simulink model "PHRI_MODEL_PROJECT"  (R2020b)
settings: Solver=VariableStepAuto  StartTime=0.0  StopTime=20  RelTol=1e-3
values from neighbouring files (symbols this model uses):
  A = [1 Ts;0 1]    [parameters.m]
  Be = 1    [parameters.m]
  beta = 2*pi*Fc*Ts / (1+2*pi*Fc*Ts)    (= 0.111635211705)    [parameters.m]
  Bh = 0.02    [parameters.m]
  Bh_hat = 0.05    [parameters.m]
  C = [1 0]    [parameters.m]
  delayCommM2S = 400    [parameters.m]
  delayCommS2M = 400    [parameters.m]
  Fc = 20    [parameters.m]
  Fc_h = 1    [parameters.m]
  Jh = 0.00002    (= 2e-05)    [parameters.m]
  k_m = 19.34    [parameters.m]
  k_s = 19.34    [parameters.m]
  Kc2v_m = 2    [parameters.m]
  Kc2v_s = 2    [parameters.m]
  Kd_h = 1.125    [parameters.m]
  Kd_m = 1.5    [parameters.m]
  Kd_s = 1.5    [parameters.m]
  Ke = 10    [parameters.m]
  Kh_hat = 1    [parameters.m]
  Kh_max = 50    [parameters.m]
  Kp_h = 1    [parameters.m]
  Kp_m = 1    [parameters.m]
  Kp_s = 1    [parameters.m]
  Kt2c_m = 1.182    [parameters.m]
  Kt2c_s = 1.182    [parameters.m]
  lArm_m = 0.1    [parameters.m]
  lArm_s = 0.1    [parameters.m]
  maxCurrent_m = 4.5    [parameters.m]
  maxCurrent_s = 4.5    [parameters.m]
  PosRef = 1    [parameters.m]
  qe = 2    [parameters.m]
  stopTime = str2double(stopTime)    [parameters.m]
  tau_m = 1.217    [parameters.m]
  tau_s = 1.217    [parameters.m]
  Ts = 0.001    [parameters.m]
  Variance = 0.0000001    (= 1e-07)    [parameters.m]
undefined symbols (not defined in the file or in its folder): DiscIntNeverNeededParam, Discrete, Time
libraries: simulink_extras x37, dspsigops x37, ctrlSharedLib x16, cstblocks x1
(part 2 of 3)

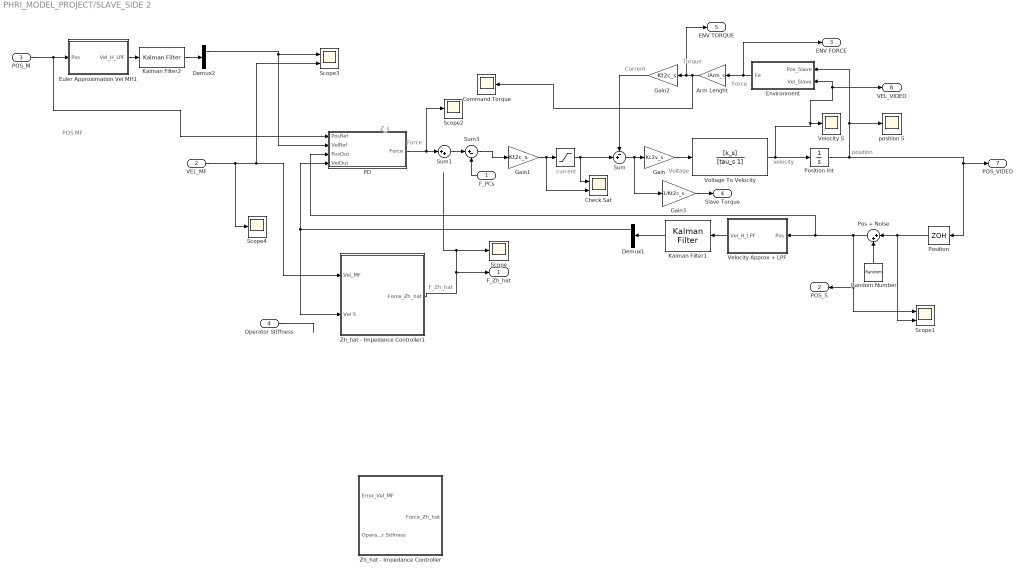
== system PHRI_MODEL_PROJECT/SLAVE_SIDE 2 ==
  note: POS MF
  note: current
  note: Force
  note: velocity
  note: position
  note: Current
  note: Voltage
  note: Torque
  note: Z_s
  note: Force
  note: F_Zh_hat
  F_PCs : Inport
  VEL_MF : Inport  Port=2
  POS_M : Inport  Port=3
  Operator Stiffness : Inport  Port=4
  " " : Saturate  UpperLimit=maxCurrent_s  LowerLimit=-maxCurrent_s
  Arm Lenght : Gain  Gain=lArm_s
  Check Sat : Scope  NumInputPorts=2
  Command Torque : Scope
  Demux1 : Demux  Outputs=2
  Demux2 : Demux  Outputs=2
  "Environment " : Subsystem
  Euler Approximation Vel MH1 : Subsystem
  Gain : Gain  Gain=Kc2v_s
  Gain1 : Gain  Gain=Kt2c_s
  Gain2 : Gain  Gain=Kt2c_s
  Gain3 : Gain  Gain=1/Kt2c_s
  Kalman Filter1 : ctrlSharedLib/Kalman Filter  TimeDomain=Discrete-Time  UseCurrentEstimator=off  ModelSource=Individual A, B, C, D matrices  ModelSourceVariable=ss(A,0,C,0)  A=A  B=1  C=C  D=0  NumberOfStates=2  NumberOfInputs=1  NumberOfOutputs=1  InitialEstimateSource=Dialog  X0=0  P0=10  UseK=off  UseGH=off  NumberOfProcessNoiseInputs=1  G=1  TimeInvariantG=on  H=0  TimeInvariantH=on  Q=0.05  TimeInvariantQ=on  R=1  TimeInvariantR=on  N=0  TimeInvariantN=on  AddInputPort=off  AddEnablePort=off  OutputEstimatedY=off  OutputP=off  Ts=Ts
  Kalman Filter2 : ctrlSharedLib/Kalman Filter  TimeDomain=Discrete-Time  UseCurrentEstimator=off  ModelSource=Individual A, B, C, D matrices  ModelSourceVariable=ss(A,0,C,0)  A=A  B=1  C=C  D=0  NumberOfStates=2  NumberOfInputs=1  NumberOfOutputs=1  InitialEstimateSource=Dialog  X0=0  P0=10  UseK=off  UseGH=off  NumberOfProcessNoiseInputs=1  G=1  TimeInvariantG=on  H=0  TimeInvariantH=on  Q=0.05  TimeInvariantQ=on  R=1  TimeInvariantR=on  N=0  TimeInvariantN=on  AddInputPort=off  AddEnablePort=off  OutputEstimatedY=off  OutputP=off  Ts=Ts
  PD : Subsystem
  Pos + Noise : Sum  Inputs=|++
  Position : ZeroOrderHold  SampleTime=Ts
  "Position Int " : Integrator
  Random Number : RandomNumber  Variance=Variance  SampleTime=Ts
  Scope : Scope
  Scope1 : Scope  NumInputPorts=2
  Scope2 : Scope
  Scope3 : Scope  NumInputPorts=2
  Scope4 : Scope
  Sum : Sum  Inputs=-+|
  Sum1 : Sum  Inputs=|++
  Sum3 : Sum  Inputs=|+-
  "Velocity Approx + LPF " : Subsystem
  Velocity S : Scope
  "Voltage To Velocity " : TransferFcn  Numerator=[k_s]  Denominator=[tau_s 1]
  Zh_hat - Impedance Controller : Subsystem
  Zh_hat - Impedance Controller1 : Subsystem
  "position S " : Scope
  F_Zh_hat : Outport
  POS_S : Outport  Port=2
  ENV FORCE : Outport  Port=3
  Slave Torque : Outport  Port=4
  ENV TORQUE : Outport  Port=5
  VEL_VIDEO : Outport  Port=6
  POS_VIDEO : Outport  Port=7
  wires:
  PD/1(Force) -> Scope2/1, Sum1/1
  "Position Int "/1 -> Position/1, POS_VIDEO/1, "position S "/1, "Environment "/1(Pos_Slave)
  Gain1/1 -> Check Sat/2, " "/1
  Gain2/1 -> Sum/1
  "Environment "/1(Fe) -> ENV FORCE/1, Arm Lenght/1
  "Voltage To Velocity "/1 -> "Position Int "/1, Velocity S/1, "Environment "/2("Vel_Slave "), VEL_VIDEO/1
  Sum/1 -> Gain3/1, Gain/1
  Gain/1 -> "Voltage To Velocity "/1
  Sum1/1 -> Sum3/1
  " "/1 -> Check Sat/1, Sum/2
  Arm Lenght/1 -> Command Torque/1, ENV TORQUE/1, Gain2/1
  Zh_hat - Impedance Controller1/1("Force_Zh_hat ") -> Scope/1, F_Zh_hat/1
  F_PCs/1 -> Sum3/2
  Operator Stiffness/1 -> ?
  VEL_MF/1 -> Scope4/1, Scope3/2, Zh_hat - Impedance Controller1/1(Vel_MF)
  Pos + Noise/1 -> PD/3(PosOut), "Velocity Approx + LPF "/1(Pos), POS_S/1, Scope1/1
  Random Number/1 -> Pos + Noise/2
  Demux1/1 -> PD/4(VelOut), Zh_hat - Impedance Controller1/2(Vel S)
  Position/1 -> Scope1/2, Pos + Noise/1
  "Velocity Approx + LPF "/1("Vel_H_LPF ") -> Kalman Filter1/1
  Kalman Filter1/1 -> Demux1/1
  Gain3/1 -> Slave Torque/1
  POS_M/1 -> PD/1(PosRef), Euler Approximation Vel MH1/1(Pos)
  Euler Approximation Vel MH1/1("Vel_H_LPF ") -> Kalman Filter2/1
  Kalman Filter2/1 -> Demux2/1
  Demux2/1 -> PD/2(VelRef), Scope3/1
  Sum3/1 -> Gain1/1

== system PHRI_MODEL_PROJECT/Velocity Approx + LPF 3 ==
  Pos : Inport
  Constant : Constant  Value=Ts  SampleTime=Ts
  Constant1 : Constant  Value=beta
  "Euler Approximation " : MATLAB Function  TreatAsAtomicUnit=on
  Unit Delay : UnitDelay  SampleTime=Ts  HasFrameUpgradeWarning=on
  Unit Delay1 : UnitDelay  SampleTime=Ts  HasFrameUpgradeWarning=on
  "Vel_H_LPF " : Outport
  wires:
  Pos/1 -> Unit Delay/1, "Euler Approximation "/3(pos)
  Constant/1 -> "Euler Approximation "/2(Ts)
  Unit Delay/1 -> "Euler Approximation "/4(posPrev)
  Unit Delay1/1 -> "Euler Approximation "/5(filteredPrev)
  "Euler Approximation "/1(filtered) -> Unit Delay1/1, "Vel_H_LPF "/1
  Constant1/1 -> "Euler Approximation "/1(beta)

== system PHRI_MODEL_PROJECT/MASTER SIDE/Intentional operator force ==
  Pos Ref : Inport
  Vel Ref : Inport  Port=2
  Pos Slave : Inport  Port=3
  Vel Slave : Inport  Port=4
  Gain : Gain  Gain=Kp_h
  Gain1 : Gain  Gain=Kd_h
  Sum : Sum
  Sum1 : Sum  Inputs=+-
  Sum2 : Sum  Inputs=+-
  "Fh_star " : Outport
  wires:
  Sum/1 -> "Fh_star "/1
  Pos Ref/1 -> Sum1/1
  Pos Slave/1 -> Sum1/2
  Vel Ref/1 -> Sum2/1
  Vel Slave/1 -> Sum2/2
  Sum1/1 -> Gain/1
  Sum2/1 -> Gain1/1
  Gain1/1 -> Sum/2
  Gain/1 -> Sum/1

== system PHRI_MODEL_PROJECT/MASTER SIDE/Operator - Dynamic model ==
  "Velocity master " : Inport
  Derivative : Derivative  CoefficientInTFapproximation=0.01
  Friction : Gain  Gain=Bh
  Inertia : Gain  Gain=Jh
  Integrator : Integrator
  "Stiffness " : Gain  Gain=Kh_hat
  Sum : Sum  Inputs=+++
  Force : Outport
  wires:
  "Velocity master "/1 -> Friction/1, Integrator/1, Derivative/1
  Derivative/1 -> Inertia/1
  Inertia/1 -> Sum/2
  Friction/1 -> Sum/1
  Sum/1 -> Force/1
  Integrator/1 -> "Stiffness "/1
  "Stiffness "/1 -> ?

== system PHRI_MODEL_PROJECT/MASTER SIDE/Velocity Approx + LPF 3 ==
  Pos : Inport
  Constant : Constant  Value=Ts  SampleTime=Ts
  Constant1 : Constant  Value=beta
  "Euler Approximation " : MATLAB Function  TreatAsAtomicUnit=on
  Unit Delay : UnitDelay  SampleTime=Ts  HasFrameUpgradeWarning=on
  Unit Delay1 : UnitDelay  SampleTime=Ts  HasFrameUpgradeWarning=on
  "Vel_H_LPF " : Outport
  wires:
  Pos/1 -> Unit Delay/1, "Euler Approximation "/3(pos)
  Constant/1 -> "Euler Approximation "/2(Ts)
  Unit Delay/1 -> "Euler Approximation "/4(posPrev)
  Unit Delay1/1 -> "Euler Approximation "/5(filteredPrev)
  "Euler Approximation "/1(filtered) -> Unit Delay1/1, "Vel_H_LPF "/1
  Constant1/1 -> "Euler Approximation "/1(beta)

== system PHRI_MODEL_PROJECT/MASTER SIDE1/Euler Approximation Vel MH2 ==
  Pos : Inport
  Clock : simulink_extras/Flip Flops/Clock  period=Ts*2
  Clock1 : simulink_extras/Flip Flops/Clock  period=Ts*2
  Constant : Constant  Value=Ts
  Constant1 : Constant  Value=beta
  "Euler Approximation " : MATLAB Function  TreatAsAtomicUnit=on
  Sample and Hold : dspsigops/Sample and Hold  trig=Rising edge  initCond=0  latchinput=on
  Sample and Hold1 : dspsigops/Sample and Hold  trig=Rising edge  initCond=0  latchinput=on
  "Vel_H_LPF " : Outport
  wires:
  Pos/1 -> Sample and Hold/1, "Euler Approximation "/3(pos)
  Constant/1 -> "Euler Approximation "/2(Ts)
  Sample and Hold/1 -> "Euler Approximation "/4(posPrev)
  Clock/1 -> Sample and Hold/Trigger
  Sample and Hold1/1 -> "Euler Approximation "/5(filteredPrev)
  "Euler Approximation "/1(filtered) -> "Vel_H_LPF "/1, Sample and Hold1/1
  Clock1/1 -> Sample and Hold1/Trigger
  Constant1/1 -> "Euler Approximation "/1(beta)

== system PHRI_MODEL_PROJECT/MASTER SIDE1/Intentional operator force ==
  Pos Ref : Inport
  Vel Ref : Inport  Port=2
  Pos Slave : Inport  Port=3
  Vel Slave : Inport  Port=4
  Gain : Gain  Gain=Kp_h
  Gain1 : Gain  Gain=Kd_h
  Sum : Sum
  Sum1 : Sum  Inputs=+-
  Sum2 : Sum  Inputs=+-
  "Fh_star " : Outport
  wires:
  Sum/1 -> "Fh_star "/1
  Pos Ref/1 -> Sum1/1
  Pos Slave/1 -> Sum1/2
  Vel Ref/1 -> Sum2/1
  Vel Slave/1 -> Sum2/2
  Sum1/1 -> Gain/1
  Sum2/1 -> Gain1/1
  Gain1/1 -> Sum/2
  Gain/1 -> Sum/1

== system PHRI_MODEL_PROJECT/MASTER SIDE1/Subsystem ==
  "Velocità " : Inport
  Derivative : Derivative  CoefficientInTFapproximation=0.01
  Friction : Gain  Gain=Bh
  Inertia : Gain  Gain=Jh
  Integrator : Integrator
  "Stiffness " : Gain  Gain=Kh_hat
  Sum : Sum  Inputs=+++
  Force : Outport
  wires:
  "Velocità "/1 -> Friction/1, Integrator/1, Derivative/1
  Derivative/1 -> Inertia/1
  Inertia/1 -> Sum/2
  Friction/1 -> Sum/1
  Sum/1 -> Force/1
  Integrator/1 -> "Stiffness "/1
  "Stiffness "/1 -> ?

== system PHRI_MODEL_PROJECT/MASTER SIDE1/Velocity Approx + LPF  ==
  Pos : Inport
  Clock : simulink_extras/Flip Flops/Clock  period=Ts*2
  Clock1 : simulink_extras/Flip Flops/Clock  period=Ts*2
  Constant : Constant  Value=Ts
  Constant1 : Constant  Value=beta
  "Euler Approximation " : MATLAB Function  TreatAsAtomicUnit=on
  Sample and Hold : dspsigops/Sample and Hold  trig=Rising edge  initCond=0  latchinput=on
  Sample and Hold1 : dspsigops/Sample and Hold  trig=Rising edge  initCond=0  latchinput=on
  "Vel_H_LPF " : Outport
  wires:
  Pos/1 -> Sample and Hold/1, "Euler Approximation "/3(pos)
  Constant/1 -> "Euler Approximation "/2(Ts)
  Sample and Hold/1 -> "Euler Approximation "/4(posPrev)
  Clock/1 -> Sample and Hold/Trigger
  Sample and Hold1/1 -> "Euler Approximation "/5(filteredPrev)
  "Euler Approximation "/1(filtered) -> "Vel_H_LPF "/1, Sample and Hold1/1
  Clock1/1 -> Sample and Hold1/Trigger
  Constant1/1 -> "Euler Approximation "/1(beta)

== system PHRI_MODEL_PROJECT/MASTER SIDE1/Virtual Coupling ==
  Pos Master : Inport
  Vel Master : Inport  Port=2
  Pos Slave : Inport  Port=3
  Vel Slave : Inport  Port=4
  Gain : Gain  Gain=Kp_m
  Gain1 : Gain  Gain=Kd_m
  Sum : Sum
  Sum1 : Sum  Inputs=-+
  Sum2 : Sum  Inputs=-+
  "F Env Virt " : Outport
  wires:
  Gain/1 -> Sum/1
  Gain1/1 -> Sum/2
  Sum2/1 -> Gain1/1
  Sum1/1 -> Gain/1
  Vel Slave/1 -> Sum2/2
  Vel Master/1 -> Sum2/1
  Pos Slave/1 -> Sum1/2
  Pos Master/1 -> Sum1/1
  Sum/1 -> "F Env Virt "/1

== system PHRI_MODEL_PROJECT/MASTER SIDE2/Intentional operator force ==
  Pos Ref : Inport
  Vel Ref : Inport  Port=2
  Pos Slave : Inport  Port=3
  Vel Slave : Inport  Port=4
  Gain : Gain  Gain=Kp_h
  Gain1 : Gain  Gain=Kd_h
  Sum : Sum
  Sum1 : Sum  Inputs=+-
  Sum2 : Sum  Inputs=+-
  "Fh_star " : Outport
  wires:
  Sum/1 -> "Fh_star "/1
  Pos Ref/1 -> Sum1/1
  Pos Slave/1 -> Sum1/2
  Vel Ref/1 -> Sum2/1
  Vel Slave/1 -> Sum2/2
  Sum1/1 -> Gain/1
  Sum2/1 -> Gain1/1
  Gain1/1 -> Sum/2
  Gain/1 -> Sum/1

== system PHRI_MODEL_PROJECT/MASTER SIDE2/Subsystem ==
  "Velocità " : Inport
  Derivative : Derivative  CoefficientInTFapproximation=0.01
  Friction : Gain  Gain=Bh
  Inertia : Gain  Gain=Jh
  Integrator : Integrator
  "Stiffness " : Gain  Gain=Kh_hat
  Sum : Sum  Inputs=+++
  Force : Outport
  wires:
  "Velocità "/1 -> Friction/1, Integrator/1, Derivative/1
  Derivative/1 -> Inertia/1
  Inertia/1 -> Sum/2
  Friction/1 -> Sum/1
  Sum/1 -> Force/1
  Integrator/1 -> "Stiffness "/1
  "Stiffness "/1 -> ?

== system PHRI_MODEL_PROJECT/MASTER SIDE2/Velocity Approx + LPF  ==
  Pos : Inport
  Clock : simulink_extras/Flip Flops/Clock  period=Ts*2
  Clock1 : simulink_extras/Flip Flops/Clock  period=Ts*2
  Constant : Constant  Value=Ts
  Constant1 : Constant  Value=beta
  "Euler Approximation " : MATLAB Function  TreatAsAtomicUnit=on
  Sample and Hold : dspsigops/Sample and Hold  trig=Rising edge  initCond=0  latchinput=on
  Sample and Hold1 : dspsigops/Sample and Hold  trig=Rising edge  initCond=0  latchinput=on
  "Vel_H_LPF " : Outport
  wires:
  Pos/1 -> Sample and Hold/1, "Euler Approximation "/3(pos)
  Constant/1 -> "Euler Approximation "/2(Ts)
  Sample and Hold/1 -> "Euler Approximation "/4(posPrev)
  Clock/1 -> Sample and Hold/Trigger
  Sample and Hold1/1 -> "Euler Approximation "/5(filteredPrev)
  "Euler Approximation "/1(filtered) -> "Vel_H_LPF "/1, Sample and Hold1/1
  Clock1/1 -> Sample and Hold1/Trigger
  Constant1/1 -> "Euler Approximation "/1(beta)

== system PHRI_MODEL_PROJECT/MASTER SIDE2/Velocity Approx + LPF 1 ==
  Pos : Inport
  Clock : simulink_extras/Flip Flops/Clock  period=Ts*2
  Clock1 : simulink_extras/Flip Flops/Clock  period=Ts*2
  Constant : Constant  Value=Ts
  Constant1 : Constant  Value=beta
  "Euler Approximation " : MATLAB Function  TreatAsAtomicUnit=on
  Sample and Hold : dspsigops/Sample and Hold  trig=Rising edge  initCond=0  latchinput=on
  Sample and Hold1 : dspsigops/Sample and Hold  trig=Rising edge  initCond=0  latchinput=on
  "Vel_H_LPF " : Outport
  wires:
  Pos/1 -> Sample and Hold/1, "Euler Approximation "/3(pos)
  Constant/1 -> "Euler Approximation "/2(Ts)
  Sample and Hold/1 -> "Euler Approximation "/4(posPrev)
  Clock/1 -> Sample and Hold/Trigger
  Sample and Hold1/1 -> "Euler Approximation "/5(filteredPrev)
  "Euler Approximation "/1(filtered) -> "Vel_H_LPF "/1, Sample and Hold1/1
  Clock1/1 -> Sample and Hold1/Trigger
  Constant1/1 -> "Euler Approximation "/1(beta)

== system PHRI_MODEL_PROJECT/MASTER SIDE2/Velocity Approx + LPF 2 ==
  Pos : Inport
  Clock : simulink_extras/Flip Flops/Clock  period=Ts*2
  Clock1 : simulink_extras/Flip Flops/Clock  period=Ts*2
  Constant : Constant  Value=Ts
  Constant1 : Constant  Value=beta
  "Euler Approximation " : MATLAB Function  TreatAsAtomicUnit=on
  Sample and Hold : dspsigops/Sample and Hold  trig=Rising edge  initCond=0  latchinput=on
  Sample and Hold1 : dspsigops/Sample and Hold  trig=Rising edge  initCond=0  latchinput=on
  "Vel_H_LPF " : Outport
  wires:
  Pos/1 -> Sample and Hold/1, "Euler Approximation "/3(pos)
  Constant/1 -> "Euler Approximation "/2(Ts)
  Sample and Hold/1 -> "Euler Approximation "/4(posPrev)
  Clock/1 -> Sample and Hold/Trigger
  Sample and Hold1/1 -> "Euler Approximation "/5(filteredPrev)
  "Euler Approximation "/1(filtered) -> "Vel_H_LPF "/1, Sample and Hold1/1
  Clock1/1 -> Sample and Hold1/Trigger
  Constant1/1 -> "Euler Approximation "/1(beta)

== system PHRI_MODEL_PROJECT/MASTER SIDE2/Velocity Approx + LPF 3 ==
  Pos : Inport
  Clock : simulink_extras/Flip Flops/Clock  period=Ts*2
  Clock1 : simulink_extras/Flip Flops/Clock  period=Ts*2
  Constant : Constant  Value=Ts
  Constant1 : Constant  Value=beta
  "Euler Approximation " : MATLAB Function  TreatAsAtomicUnit=on
  Sample and Hold : dspsigops/Sample and Hold  trig=Rising edge  initCond=0  latchinput=on
  Sample and Hold1 : dspsigops/Sample and Hold  trig=Rising edge  initCond=0  latchinput=on
  "Vel_H_LPF " : Outport
  wires:
  Pos/1 -> Sample and Hold/1, "Euler Approximation "/3(pos)
  Constant/1 -> "Euler Approximation "/2(Ts)
  Sample and Hold/1 -> "Euler Approximation "/4(posPrev)
  Clock/1 -> Sample and Hold/Trigger
  Sample and Hold1/1 -> "Euler Approximation "/5(filteredPrev)
  "Euler Approximation "/1(filtered) -> "Vel_H_LPF "/1, Sample and Hold1/1
  Clock1/1 -> Sample and Hold1/Trigger
  Constant1/1 -> "Euler Approximation "/1(beta)

== system PHRI_MODEL_PROJECT/POPC - Master Side/PC - Master side ==
  E_PO - Master : Inport
  "Velocity Master " : Inport  Port=2
  E_POm : Scope
  E_POm1 : Scope
  PASSIVE CONTROLLER PCm : MATLAB Function  TreatAsAtomicUnit=on
  Unit Delay : UnitDelay  SampleTime=Ts  HasFrameUpgradeWarning=on
  dt : Constant  Value=Ts
  ALPHA : Outport
  Energy PCm : Outport  Port=2
  wires:
  Unit Delay/1 -> Energy PCm/1, PASSIVE CONTROLLER PCm/4(E_PCm_prev)
  dt/1 -> PASSIVE CONTROLLER PCm/2(Ts)
  E_PO - Master/1 -> E_POm/1, PASSIVE CONTROLLER PCm/1(E_POm)
  PASSIVE CONTROLLER PCm/1(E_PCm) -> Unit Delay/1
  PASSIVE CONTROLLER PCm/2(alpha_m) -> E_POm1/1, ALPHA/1
  "Velocity Master "/1 -> PASSIVE CONTROLLER PCm/3(v_m)

== system PHRI_MODEL_PROJECT/POPC - Master Side/PO Input - Slave to Master (Cause) ==
  Force_Env : Inport
  Velocity Master Delayed : Inport  Port=2
  E_Rin : Scope
  PASSIVE OBSERVER S2M E Right INPUT : Subsystem
  Input Energy : Outport
  wires:
  PASSIVE OBSERVER S2M E Right INPUT/1(E-Rin) -> Input Energy/1, E_Rin/1
  Velocity Master Delayed/1 -> PASSIVE OBSERVER S2M E Right INPUT/2("Vel_M ")
  Force_Env/1 -> PASSIVE OBSERVER S2M E Right INPUT/1(Env_Force)

== system PHRI_MODEL_PROJECT/POPC - Master Side/PO Output - Master to Slave (Effect) ==
  note: E Left Out
  Velocity Master : Inport
  Force Env Delayed : Inport  Port=2
  E_Lout : Scope
  PASSIVE OBSERVER M2S E Left OUTPUT : Subsystem
  Output energy : Outport
  wires:
  Velocity Master/1 -> PASSIVE OBSERVER M2S E Left OUTPUT/1(Velocity Master)
  PASSIVE OBSERVER M2S E Left OUTPUT/1(E-Lout) -> Output energy/1, E_Lout/1
  Force Env Delayed/1 -> PASSIVE OBSERVER M2S E Left OUTPUT/2(Force Env Delayed)

== system PHRI_MODEL_PROJECT/POPC - Master Side1/PC - Master side ==
  E_PO - Master : Inport
  "Velocity Master " : Inport  Port=2
  Clock : simulink_extras/Flip Flops/Clock  period=Ts*2
  E_POm : Scope
  PASSIVE CONTROLLER PCm : MATLAB Function  TreatAsAtomicUnit=on
  Sample and Hold : dspsigops/Sample and Hold  trig=Rising edge  initCond=0  latchinput=on
  dt : Constant  Value=Ts
  ALPHA : Outport
  Energy PCm : Outport  Port=2
  wires:
  Sample and Hold/1 -> PASSIVE CONTROLLER PCm/4(E_PCm_prev)
  dt/1 -> PASSIVE CONTROLLER PCm/2(dt)
  E_PO - Master/1 -> E_POm/1, PASSIVE CONTROLLER PCm/1(E_POm)
  Clock/1 -> Sample and Hold/Trigger
  PASSIVE CONTROLLER PCm/1(E_PCm) -> Sample and Hold/1, Energy PCm/1
  PASSIVE CONTROLLER PCm/2(alpha_m) -> ALPHA/1
  "Velocity Master "/1 -> PASSIVE CONTROLLER PCm/3(v_m)

== system PHRI_MODEL_PROJECT/POPC - Master Side1/PO Input - Slave to Master (Cause) ==
  Force_Env : Inport
  Velocity Master Delayed : Inport  Port=2
  E_Rin : Scope
  PASSIVE OBSERVER S2M E Right INPUT : Subsystem
  Input Energy : Outport
  wires:
  PASSIVE OBSERVER S2M E Right INPUT/1(E-Rin) -> Input Energy/1, E_Rin/1
  Velocity Master Delayed/1 -> PASSIVE OBSERVER S2M E Right INPUT/2("Vel_M ")
  Force_Env/1 -> PASSIVE OBSERVER S2M E Right INPUT/1(Env_Force)

== system PHRI_MODEL_PROJECT/POPC - Master Side1/PO Output - Master to Slave (Effect) ==
  note: E Left Out
  Velocity Master : Inport
  Force Env Delayed : Inport  Port=2
  E_Lout : Scope
  PASSIVE OBSERVER M2S E Left OUTPUT : Subsystem
  Output energy : Outport
  wires:
  Velocity Master/1 -> PASSIVE OBSERVER M2S E Left OUTPUT/1(Velocity Master)
  PASSIVE OBSERVER M2S E Left OUTPUT/1(E-Lout) -> Output energy/1, E_Lout/1
  Force Env Delayed/1 -> PASSIVE OBSERVER M2S E Left OUTPUT/2(Force Env Delayed)

== system PHRI_MODEL_PROJECT/POPC - Master Side2/PC - Master side ==
  E_PO - Master : Inport
  "Velocity Master " : Inport  Port=2
  Clock : simulink_extras/Flip Flops/Clock  period=Ts*2
  E_POm : Scope
  PASSIVE CONTROLLER PCm : MATLAB Function  TreatAsAtomicUnit=on
  Sample and Hold : dspsigops/Sample and Hold  trig=Rising edge  initCond=0  latchinput=on
  dt : Constant  Value=Ts
  ALPHA : Outport
  Energy PCm : Outport  Port=2
  wires:
  Sample and Hold/1 -> PASSIVE CONTROLLER PCm/4(E_PCm_prev)
  dt/1 -> PASSIVE CONTROLLER PCm/2(dt)
  E_PO - Master/1 -> E_POm/1, PASSIVE CONTROLLER PCm/1(E_POm)
  Clock/1 -> Sample and Hold/Trigger
  PASSIVE CONTROLLER PCm/1(E_PCm) -> Sample and Hold/1, Energy PCm/1
  PASSIVE CONTROLLER PCm/2(alpha_m) -> ALPHA/1
  "Velocity Master "/1 -> PASSIVE CONTROLLER PCm/3(v_m)

== system PHRI_MODEL_PROJECT/POPC - Master Side2/PO Input - Slave to Master (Cause) ==
  Force_Env : Inport
  Velocity Master Delayed : Inport  Port=2
  E_Rin : Scope
  PASSIVE OBSERVER S2M E Right INPUT : Subsystem
  Input Energy : Outport
  wires:
  PASSIVE OBSERVER S2M E Right INPUT/1(E-Rin) -> Input Energy/1, E_Rin/1
  Velocity Master Delayed/1 -> PASSIVE OBSERVER S2M E Right INPUT/2("Vel_M ")
  Force_Env/1 -> PASSIVE OBSERVER S2M E Right INPUT/1(Env_Force)

== system PHRI_MODEL_PROJECT/POPC - Master Side2/PO Output - Master to Slave (Effect) ==
  note: E Left Out
  Velocity Master : Inport
  Force Env Delayed : Inport  Port=2
  E_Lout : Scope
  PASSIVE OBSERVER M2S E Left OUTPUT : Subsystem
  Output energy : Outport
  wires:
  Velocity Master/1 -> PASSIVE OBSERVER M2S E Left OUTPUT/1(Velocity Master)
  PASSIVE OBSERVER M2S E Left OUTPUT/1(E-Lout) -> Output energy/1, E_Lout/1
  Force Env Delayed/1 -> PASSIVE OBSERVER M2S E Left OUTPUT/2(Force Env Delayed)

== system PHRI_MODEL_PROJECT/POPC - Slave Side/PASSIVE OBSERVER Left Input ==
  Force Env Delayed : Inport
  Velocity Master : Inport  Port=2
  Add : Sum
  Product : Product
  Unit Delay : UnitDelay  SampleTime=Ts  HasFrameUpgradeWarning=on
  E-Lin : Outport
  wires:
  Velocity Master/1 -> Product/1
  Force Env Delayed/1 -> Product/2
  Product/1 -> Add/2
  Unit Delay/1 -> Add/1
  Add/1 -> Unit Delay/1, E-Lin/1

== system PHRI_MODEL_PROJECT/POPC - Slave Side/PASSIVE OBSERVER Right Output ==
  Force Env : Inport
  Velocity Master delayed : Inport  Port=2
  Add : Sum
  Product : Product
  Unit Delay : UnitDelay  SampleTime=Ts  HasFrameUpgradeWarning=on
  E-Rout : Outport
  wires:
  Velocity Master delayed/1 -> Product/1
  Force Env/1 -> Product/2
  Product/1 -> Add/2
  Unit Delay/1 -> Add/1
  Add/1 -> Unit Delay/1, E-Rout/1

== system PHRI_MODEL_PROJECT/POPC - Slave Side/PC Slave ==
  Energy POs : Inport
  Velocity Slave : Inport  Port=2
  Clock1 : simulink_extras/Flip Flops/Clock  period=Ts
  PASSIVE CONTROLLER PCs : MATLAB Function  TreatAsAtomicUnit=on
  Sample and Hold1 : dspsigops/Sample and Hold  trig=Rising edge  initCond=0  latchinput=on
  Scope : Scope
  Scope1 : Scope  NumInputPorts=3
  Unit Delay : UnitDelay  SampleTime=Ts  HasFrameUpgradeWarning=on
  dt1 : Constant  Value=Ts
  Energy PC : Outport
  ALPHA : Outport  Port=2
  wires:
  PASSIVE CONTROLLER PCs/1(E_PCs) -> Unit Delay/1, Scope1/3
  dt1/1 -> PASSIVE CONTROLLER PCs/3(Ts)
  PASSIVE CONTROLLER PCs/2(alpha_s) -> ALPHA/1
  Energy POs/1 -> Scope1/1, Scope/1, PASSIVE CONTROLLER PCs/2(E_POs)
  Unit Delay/1 -> Scope1/2, Energy PC/1, PASSIVE CONTROLLER PCs/1(E_PCs_prev)
  Velocity Slave/1 -> PASSIVE CONTROLLER PCs/4(v_s)
  Clock1/1 -> Sample and Hold1/Trigger

== system PHRI_MODEL_PROJECT/POPC - Slave Side1/PASSIVE OBSERVER Left Input ==
  Force Impedance Delayed : Inport
  Velocity MF : Inport  Port=2
  Add : Sum
  Clock : simulink_extras/Flip Flops/Clock  period=Ts*2
  Product : Product
  Sample and Hold : dspsigops/Sample and Hold  trig=Rising edge  initCond=0  latchinput=on
  E-Lin : Outport
  wires:
  Velocity MF/1 -> Product/1
  Force Impedance Delayed/1 -> Product/2
  Product/1 -> Add/2
  Sample and Hold/1 -> Add/1
  Add/1 -> Sample and Hold/1, E-Lin/1
  Clock/1 -> Sample and Hold/Trigger

== system PHRI_MODEL_PROJECT/POPC - Slave Side1/PASSIVE OBSERVER Right Output ==
  Force Impedence : Inport
  Velocity MF delayed : Inport  Port=2
  Add : Sum
  Clock : simulink_extras/Flip Flops/Clock  period=Ts*2
  Product : Product
  Sample and Hold : dspsigops/Sample and Hold  trig=Rising edge  initCond=0  latchinput=on
  E-Rout : Outport
  wires:
  Velocity MF delayed/1 -> Product/1
  Force Impedence/1 -> Product/2
  Product/1 -> Add/2
  Sample and Hold/1 -> Add/1
  Add/1 -> Sample and Hold/1, E-Rout/1
  Clock/1 -> Sample and Hold/Trigger

== system PHRI_MODEL_PROJECT/POPC - Slave Side1/PC Slave ==
  Energy POs : Inport
  Velocity Slave : Inport  Port=2
  Clock1 : simulink_extras/Flip Flops/Clock  period=Ts*2
  PASSIVE CONTROLLER PCs : MATLAB Function  TreatAsAtomicUnit=on
  Sample and Hold1 : dspsigops/Sample and Hold  trig=Rising edge  initCond=0  latchinput=on
  dt1 : Constant  Value=Ts
  Energy PC : Outport
  ALPHA : Outport  Port=2
  wires:
  PASSIVE CONTROLLER PCs/1(E_PCs) -> Sample and Hold1/1
  dt1/1 -> PASSIVE CONTROLLER PCs/3(Ts)
  PASSIVE CONTROLLER PCs/2(alpha_s) -> ALPHA/1
  Energy POs/1 -> PASSIVE CONTROLLER PCs/2(E_POs)
  Clock1/1 -> Sample and Hold1/Trigger
  Sample and Hold1/1 -> Energy PC/1, PASSIVE CONTROLLER PCs/1(E_PCs_prev)
  Velocity Slave/1 -> PASSIVE CONTROLLER PCs/4(v_s)

== system PHRI_MODEL_PROJECT/POPC - Slave Side2/PASSIVE OBSERVER Left Input ==
  Force Impedance Delayed : Inport
  Velocity MF : Inport  Port=2
  Add : Sum
  Clock : simulink_extras/Flip Flops/Clock  period=Ts*2
  Product : Product
  Sample and Hold : dspsigops/Sample and Hold  trig=Rising edge  initCond=0  latchinput=on
  E-Lin : Outport
  wires:
  Velocity MF/1 -> Product/1
  Force Impedance Delayed/1 -> Product/2
  Product/1 -> Add/2
  Sample and Hold/1 -> Add/1
  Add/1 -> Sample and Hold/1, E-Lin/1
  Clock/1 -> Sample and Hold/Trigger

== system PHRI_MODEL_PROJECT/POPC - Slave Side2/PASSIVE OBSERVER Right Output ==
  Force Impedence : Inport
  Velocity MF delayed : Inport  Port=2
  Add : Sum
  Clock : simulink_extras/Flip Flops/Clock  period=Ts*2
  Product : Product
  Sample and Hold : dspsigops/Sample and Hold  trig=Rising edge  initCond=0  latchinput=on
  E-Rout : Outport
  wires:
  Velocity MF delayed/1 -> Product/1
  Force Impedence/1 -> Product/2
  Product/1 -> Add/2
  Sample and Hold/1 -> Add/1
  Add/1 -> Sample and Hold/1, E-Rout/1
  Clock/1 -> Sample and Hold/Trigger

== system PHRI_MODEL_PROJECT/POPC - Slave Side2/PC Slave ==
  Energy POs : Inport
  Velocity Slave : Inport  Port=2
  Clock1 : simulink_extras/Flip Flops/Clock  period=Ts*2
  PASSIVE CONTROLLER PCs : MATLAB Function  TreatAsAtomicUnit=on
  Sample and Hold1 : dspsigops/Sample and Hold  trig=Rising edge  initCond=0  latchinput=on
  dt1 : Constant  Value=Ts
  Energy PC : Outport
  ALPHA : Outport  Port=2
  wires:
  PASSIVE CONTROLLER PCs/1(E_PCs) -> Sample and Hold1/1
  dt1/1 -> PASSIVE CONTROLLER PCs/3(Ts)
  PASSIVE CONTROLLER PCs/2(alpha_s) -> ALPHA/1
  Energy POs/1 -> PASSIVE CONTROLLER PCs/2(E_POs)
  Clock1/1 -> Sample and Hold1/Trigger
  Sample and Hold1/1 -> Energy PC/1, PASSIVE CONTROLLER PCs/1(E_PCs_prev)
  Velocity Slave/1 -> PASSIVE CONTROLLER PCs/4(v_s)

== system PHRI_MODEL_PROJECT/SLAVE_SIDE /Environment  ==
  Pos_Slave : Inport
  "Vel_Slave " : Inport  Port=2
  Environment Behaviour : MATLAB Function  TreatAsAtomicUnit=on
  Environment Position : Constant  Value=qe
  Stiffness : Constant  Value=Ke
  Viscous Friction : Constant  Value=Be
  Fe : Outport
  wires:
  Pos_Slave/1 -> Environment Behaviour/1(x_s)
  "Vel_Slave "/1 -> Environment Behaviour/2(dot_x_s)
  Environment Position/1 -> Environment Behaviour/3(qe)
  Viscous Friction/1 -> Environment Behaviour/4(Be)
  Stiffness/1 -> Environment Behaviour/5(Ke)
  Environment Behaviour/1(Fe) -> Fe/1

== system PHRI_MODEL_PROJECT/SLAVE_SIDE /PD ==
  PosRef : Inport
  VelRef : Inport  Port=2
  PosOut : Inport  Port=3
  VelOut : Inport  Port=4
  Gain : Gain  Gain=Kd_s
  Gain1 : Gain  Gain=Kp_s
  Sum : Sum  Inputs=|+-
  Sum1 : Sum  Inputs=|+-
  Sum2 : Sum
  Torque : Outport
  wires:
  PosRef/1 -> Sum/1
  PosOut/1 -> Sum/2
  VelRef/1 -> Sum1/1
  VelOut/1 -> Sum1/2
  Sum1/1 -> Gain/1
  Sum/1 -> Gain1/1
  Gain1/1 -> Sum2/1
  Gain/1 -> Sum2/2
  Sum2/1 -> Torque/1

== system PHRI_MODEL_PROJECT/SLAVE_SIDE /Velocity Approx + LPF 1 ==
  Pos : Inport
  Constant : Constant  Value=Ts
  Constant1 : Constant  Value=beta
  "Euler Approximation " : MATLAB Function  TreatAsAtomicUnit=on
  Unit Delay : UnitDelay  SampleTime=Ts  HasFrameUpgradeWarning=on
  Unit Delay1 : UnitDelay  SampleTime=Ts  HasFrameUpgradeWarning=on
  "Vel_H_LPF " : Outport
  wires:
  Constant1/1 -> "Euler Approximation "/1(beta)
  "Euler Approximation "/1(filtered) -> Unit Delay1/1, "Vel_H_LPF "/1
  Unit Delay1/1 -> "Euler Approximation "/5(filteredPrev)
  Unit Delay/1 -> "Euler Approximation "/4(posPrev)
  Constant/1 -> "Euler Approximation "/2(Ts)
  Pos/1 -> Unit Delay/1, "Euler Approximation "/3(pos)

== system PHRI_MODEL_PROJECT/SLAVE_SIDE /Velocity Approx + LPF 3 ==
  Pos : Inport
  Constant : Constant  Value=Ts  SampleTime=Ts
  Constant1 : Constant  Value=beta
  "Euler Approximation " : MATLAB Function  TreatAsAtomicUnit=on
  Unit Delay : UnitDelay  SampleTime=Ts  HasFrameUpgradeWarning=on
  Unit Delay1 : UnitDelay  SampleTime=Ts  HasFrameUpgradeWarning=on
  "Vel_H_LPF " : Outport
  wires:
  Pos/1 -> Unit Delay/1, "Euler Approximation "/3(pos)
  Constant/1 -> "Euler Approximation "/2(Ts)
  Unit Delay/1 -> "Euler Approximation "/4(posPrev)
  Unit Delay1/1 -> "Euler Approximation "/5(filteredPrev)
  "Euler Approximation "/1(filtered) -> Unit Delay1/1, "Vel_H_LPF "/1
  Constant1/1 -> "Euler Approximation "/1(beta)

== system PHRI_MODEL_PROJECT/SLAVE_SIDE 1/Environment  ==
  Pos_Slave : Inport
  "Vel_Slave " : Inport  Port=2
  Environment Behaviour : MATLAB Function  TreatAsAtomicUnit=on
  Environment Position : Constant  Value=qe
  Stiffness : Constant  Value=Ke
  Viscous Friction : Constant  Value=Be
  Fe : Outport
  wires:
  Pos_Slave/1 -> Environment Behaviour/1(x_s)
  "Vel_Slave "/1 -> Environment Behaviour/2(dot_x_s)
  Environment Position/1 -> Environment Behaviour/3(qe)
  Viscous Friction/1 -> Environment Behaviour/4(Be)
  Stiffness/1 -> Environment Behaviour/5(Ke)
  Environment Behaviour/1(Fe) -> Fe/1

== system PHRI_MODEL_PROJECT/SLAVE_SIDE 1/Euler Approximation Vel MH1 ==
  Pos : Inport
  Clock : simulink_extras/Flip Flops/Clock  period=Ts*2
  Clock1 : simulink_extras/Flip Flops/Clock  period=Ts*2
  Constant : Constant  Value=Ts
  Constant1 : Constant  Value=beta
  "Euler Approximation " : MATLAB Function  TreatAsAtomicUnit=on
  Sample and Hold : dspsigops/Sample and Hold  trig=Rising edge  initCond=0  latchinput=on
  Sample and Hold1 : dspsigops/Sample and Hold  trig=Rising edge  initCond=0  latchinput=on
  "Vel_H_LPF " : Outport
  wires:
  Constant1/1 -> "Euler Approximation "/1(beta)
  Clock1/1 -> Sample and Hold1/Trigger
  "Euler Approximation "/1(filtered) -> Sample and Hold1/1, "Vel_H_LPF "/1
  Sample and Hold1/1 -> "Euler Approximation "/5(filteredPrev)
  Clock/1 -> Sample and Hold/Trigger
  Sample and Hold/1 -> "Euler Approximation "/4(posPrev)
  Constant/1 -> "Euler Approximation "/2(Ts)
  Pos/1 -> "Euler Approximation "/3(pos), Sample and Hold/1

== system PHRI_MODEL_PROJECT/SLAVE_SIDE 1/PD ==
  PosRef : Inport
  VelRef : Inport  Port=2
  PosOut : Inport  Port=3
  VelOut : Inport  Port=4
  Gain : Gain  Gain=Kd_s
  Gain1 : Gain  Gain=Kp_s
  Sum : Sum  Inputs=|+-
  Sum1 : Sum  Inputs=|+-
  Sum2 : Sum
  Force : Outport
  wires:
  PosRef/1 -> Sum/1
  PosOut/1 -> Sum/2
  VelRef/1 -> Sum1/1
  VelOut/1 -> Sum1/2
  Sum1/1 -> Gain/1
  Sum/1 -> Gain1/1
  Gain1/1 -> Sum2/1
  Gain/1 -> Sum2/2
  Sum2/1 -> Force/1

== system PHRI_MODEL_PROJECT/SLAVE_SIDE 1/Velocity Approx + LPF  ==
  Pos : Inport
  Clock : simulink_extras/Flip Flops/Clock  period=Ts*2
  Clock1 : simulink_extras/Flip Flops/Clock  period=Ts*2
  Constant : Constant  Value=Ts
  Constant1 : Constant  Value=beta
  "Euler Approximation " : MATLAB Function  TreatAsAtomicUnit=on
  Sample and Hold : dspsigops/Sample and Hold  trig=Rising edge  initCond=0  latchinput=on
  Sample and Hold1 : dspsigops/Sample and Hold  trig=Rising edge  initCond=0  latchinput=on
  "Vel_H_LPF " : Outport
  wires:
  Pos/1 -> Sample and Hold/1, "Euler Approximation "/3(pos)
  Constant/1 -> "Euler Approximation "/2(Ts)
  Sample and Hold/1 -> "Euler Approximation "/4(posPrev)
  Clock/1 -> Sample and Hold/Trigger
  Sample and Hold1/1 -> "Euler Approximation "/5(filteredPrev)
  "Euler Approximation "/1(filtered) -> "Vel_H_LPF "/1, Sample and Hold1/1
  Clock1/1 -> Sample and Hold1/Trigger
  Constant1/1 -> "Euler Approximation "/1(beta)

== system PHRI_MODEL_PROJECT/SLAVE_SIDE 1/ZCs - Impedance Controller ==
  Error_Vel_MF : Inport
  Discrete-Time Integrator : DiscreteIntegrator  SampleTime=Ts  ICPrevOutput=DiscIntNeverNeededParam  ICPrevScaledInput=DiscIntNeverNeededParam
  Gain : Gain  Gain=Kh_hat
  "Force_Zh_hat " : Outport
  wires:
  Error_Vel_MF/1 -> Discrete-Time Integrator/1
  Gain/1 -> "Force_Zh_hat "/1
  Discrete-Time Integrator/1 -> Gain/1

== system PHRI_MODEL_PROJECT/SLAVE_SIDE 2/Environment  ==
  Pos_Slave : Inport
  "Vel_Slave " : Inport  Port=2
  Environment Behaviour : MATLAB Function  TreatAsAtomicUnit=on
  Environment Position : Constant  Value=qe
  Stiffness : Constant  Value=Ke
  Viscous Friction : Constant  Value=Be
  Fe : Outport
  wires:
  Pos_Slave/1 -> Environment Behaviour/1(x_s)
  "Vel_Slave "/1 -> Environment Behaviour/2(dot_x_s)
  Environment Position/1 -> Environment Behaviour/3(qe)
  Viscous Friction/1 -> Environment Behaviour/4(Be)
  Stiffness/1 -> Environment Behaviour/5(Ke)
  Environment Behaviour/1(Fe) -> Fe/1

== system PHRI_MODEL_PROJECT/SLAVE_SIDE 2/Euler Approximation Vel MH1 ==
  Pos : Inport
  Clock : simulink_extras/Flip Flops/Clock  period=Ts*2
  Clock1 : simulink_extras/Flip Flops/Clock  period=Ts*2
  Constant : Constant  Value=Ts
  Constant1 : Constant  Value=beta
  "Euler Approximation " : MATLAB Function  TreatAsAtomicUnit=on
  Sample and Hold : dspsigops/Sample and Hold  trig=Rising edge  initCond=0  latchinput=on
  Sample and Hold1 : dspsigops/Sample and Hold  trig=Rising edge  initCond=0  latchinput=on
  "Vel_H_LPF " : Outport
  wires:
  Constant1/1 -> "Euler Approximation "/1(beta)
  Clock1/1 -> Sample and Hold1/Trigger
  "Euler Approximation "/1(filtered) -> Sample and Hold1/1, "Vel_H_LPF "/1
  Sample and Hold1/1 -> "Euler Approximation "/5(filteredPrev)
  Clock/1 -> Sample and Hold/Trigger
  Sample and Hold/1 -> "Euler Approximation "/4(posPrev)
  Constant/1 -> "Euler Approximation "/2(Ts)
  Pos/1 -> "Euler Approximation "/3(pos), Sample and Hold/1

== system PHRI_MODEL_PROJECT/SLAVE_SIDE 2/PD ==
  PosRef : Inport
  VelRef : Inport  Port=2
  PosOut : Inport  Port=3
  VelOut : Inport  Port=4
  Gain : Gain  Gain=Kd_s
  Gain1 : Gain  Gain=Kp_s
  Sum : Sum  Inputs=|+-
  Sum1 : Sum  Inputs=|+-
  Sum2 : Sum
  Force : Outport
  wires:
  PosRef/1 -> Sum/1
  PosOut/1 -> Sum/2
  VelRef/1 -> Sum1/1
  VelOut/1 -> Sum1/2
  Sum1/1 -> Gain/1
  Sum/1 -> Gain1/1
  Gain1/1 -> Sum2/1
  Gain/1 -> Sum2/2
  Sum2/1 -> Force/1

== system PHRI_MODEL_PROJECT/SLAVE_SIDE 2/Velocity Approx + LPF  ==
  Pos : Inport
  Clock : simulink_extras/Flip Flops/Clock  period=Ts*2
  Clock1 : simulink_extras/Flip Flops/Clock  period=Ts*2
  Constant : Constant  Value=Ts
  Constant1 : Constant  Value=beta
  "Euler Approximation " : MATLAB Function  TreatAsAtomicUnit=on
  Sample and Hold : dspsigops/Sample and Hold  trig=Rising edge  initCond=0  latchinput=on
  Sample and Hold1 : dspsigops/Sample and Hold  trig=Rising edge  initCond=0  latchinput=on
  "Vel_H_LPF " : Outport
  wires:
  Pos/1 -> Sample and Hold/1, "Euler Approximation "/3(pos)
  Constant/1 -> "Euler Approximation "/2(Ts)
  Sample and Hold/1 -> "Euler Approximation "/4(posPrev)
  Clock/1 -> Sample and Hold/Trigger
  Sample and Hold1/1 -> "Euler Approximation "/5(filteredPrev)
  "Euler Approximation "/1(filtered) -> "Vel_H_LPF "/1, Sample and Hold1/1
  Clock1/1 -> Sample and Hold1/Trigger
  Constant1/1 -> "Euler Approximation "/1(beta)

== system PHRI_MODEL_PROJECT/SLAVE_SIDE 2/Zh_hat - Impedance Controller ==
  Error_Vel_MF : Inport
  Operator Stifness : Inport  Port=2
  Discrete-Time Integrator1 : DiscreteIntegrator  SampleTime=Ts  ICPrevOutput=DiscIntNeverNeededParam  ICPrevScaledInput=DiscIntNeverNeededParam
  Gain : Gain  Gain=Bh
  Gain1 : Gain  Gain=Kh_hat
  Integrator : Integrator
  Product : Product
  Sum : Sum
  "Force_Zh_hat " : Outport
  wires:
  Error_Vel_MF/1 -> Integrator/1, Gain/1
  Gain/1 -> Sum/1
  Gain1/1 -> Sum/2
  Sum/1 -> "Force_Zh_hat "/1
  Operator Stifness/1 -> ?
  Integrator/1 -> Gain1/1

== system PHRI_MODEL_PROJECT/SLAVE_SIDE 2/Zh_hat - Impedance Controller1 ==
  Vel_MF : Inport
  Vel S : Inport  Port=2
  Discrete-Time Integrator : DiscreteIntegrator  SampleTime=Ts  ICPrevOutput=DiscIntNeverNeededParam  ICPrevScaledInput=DiscIntNeverNeededParam
  Gain : Gain  Gain=Bh_hat
  Gain1 : Gain  Gain=Kh_hat
  Sum : Sum
  Sum1 : Sum  Inputs=|+-
  "Force_Zh_hat " : Outport
  wires:
  Discrete-Time Integrator/1 -> Gain1/1
  Sum/1 -> "Force_Zh_hat "/1
  Gain1/1 -> Sum/2
  Gain/1 -> Sum/1
  Vel_MF/1 -> Sum1/1
  Sum1/1 -> Gain/1, Discrete-Time Integrator/1
  Vel S/1 -> Sum1/2

== system PHRI_MODEL_PROJECT/POPC - Master Side/PO Input - Slave to Master (Cause)/PASSIVE OBSERVER S2M E Right INPUT ==
  Env_Force : Inport
  "Vel_M " : Inport  Port=2
  Product : Product
  Sum : Sum
  Unit Delay : UnitDelay  SampleTime=Ts  HasFrameUpgradeWarning=on
  E-Rin : Outport
  wires:
  Env_Force/1 -> Product/1
  "Vel_M "/1 -> Product/2
  Product/1 -> Sum/2
  Sum/1 -> Unit Delay/1, E-Rin/1
  Unit Delay/1 -> Sum/1

== system PHRI_MODEL_PROJECT/POPC - Master Side/PO Output - Master to Slave (Effect)/PASSIVE OBSERVER M2S E Left OUTPUT ==
  Velocity Master : Inport
  Force Env Delayed : Inport  Port=2
  Product : Product
  Sum : Sum
  Unit Delay : UnitDelay  SampleTime=Ts  HasFrameUpgradeWarning=on
  E-Lout : Outport
  wires:
  Velocity Master/1 -> Product/1
  Force Env Delayed/1 -> Product/2
  Product/1 -> Sum/2
  Sum/1 -> Unit Delay/1, E-Lout/1
  Unit Delay/1 -> Sum/1

== system PHRI_MODEL_PROJECT/POPC - Master Side1/PO Input - Slave to Master (Cause)/PASSIVE OBSERVER S2M E Right INPUT ==
  Env_Force : Inport
  "Vel_M " : Inport  Port=2
  Clock : simulink_extras/Flip Flops/Clock  period=Ts*2
  Product : Product
  Sample and Hold : dspsigops/Sample and Hold  trig=Rising edge  initCond=0  latchinput=on
  Sum : Sum
  E-Rin : Outport
  wires:
  Env_Force/1 -> Product/1
  "Vel_M "/1 -> Product/2
  Product/1 -> Sum/2
  Sum/1 -> Sample and Hold/1, E-Rin/1
  Sample and Hold/1 -> Sum/1
  Clock/1 -> Sample and Hold/Trigger

== system PHRI_MODEL_PROJECT/POPC - Master Side1/PO Output - Master to Slave (Effect)/PASSIVE OBSERVER M2S E Left OUTPUT ==
  Velocity Master : Inport
  Force Env Delayed : Inport  Port=2
  Clock : simulink_extras/Flip Flops/Clock  period=Ts*2
  Product : Product
  Sample and Hold : dspsigops/Sample and Hold  trig=Rising edge  initCond=0  latchinput=on
  Sum : Sum
  E-Lout : Outport
  wires:
  Velocity Master/1 -> Product/1
  Force Env Delayed/1 -> Product/2
  Product/1 -> Sum/2
  Sample and Hold/1 -> Sum/1
  Sum/1 -> Sample and Hold/1, E-Lout/1
  Clock/1 -> Sample and Hold/Trigger

== system PHRI_MODEL_PROJECT/POPC - Master Side2/PO Input - Slave to Master (Cause)/PASSIVE OBSERVER S2M E Right INPUT ==
  Env_Force : Inport
  "Vel_M " : Inport  Port=2
  Clock : simulink_extras/Flip Flops/Clock  period=Ts*2
  Product : Product
  Sample and Hold : dspsigops/Sample and Hold  trig=Rising edge  initCond=0  latchinput=on
  Sum : Sum
  E-Rin : Outport
  wires:
  Env_Force/1 -> Product/1
  "Vel_M "/1 -> Product/2
  Product/1 -> Sum/2
  Sum/1 -> Sample and Hold/1, E-Rin/1
  Sample and Hold/1 -> Sum/1
  Clock/1 -> Sample and Hold/Trigger

== system PHRI_MODEL_PROJECT/POPC - Master Side2/PO Output - Master to Slave (Effect)/PASSIVE OBSERVER M2S E Left OUTPUT ==
  Velocity Master : Inport
  Force Env Delayed : Inport  Port=2
  Clock : simulink_extras/Flip Flops/Clock  period=Ts*2
  Product : Product
  Sample and Hold : dspsigops/Sample and Hold  trig=Rising edge  initCond=0  latchinput=on
  Sum : Sum
  E-Lout : Outport
  wires:
  Velocity Master/1 -> Product/1
  Force Env Delayed/1 -> Product/2
  Product/1 -> Sum/2
  Sample and Hold/1 -> Sum/1
  Sum/1 -> Sample and Hold/1, E-Lout/1
  Clock/1 -> Sample and Hold/Trigger

== matlab function PHRI_MODEL_PROJECT/Velocity Approx + LPF 3/Euler Approximation  ==
  data: beta input; Ts input; filtered output; pos input; posPrev input; filteredPrev input
function filtered = EulApprox(beta, Ts, pos, posPrev, filteredPrev)

eul= (pos - posPrev)/Ts;
filtered = beta*eul + (1-beta)*filteredPrev;

== matlab function PHRI_MODEL_PROJECT/POPC - Master Side/PC - Master side/PASSIVE CONTROLLER PCm ==
  data: E_POm input; E_PCm output; Ts input; v_m input; E_PCm_prev input; alpha_m output
function [E_PCm, alpha_m]= PC_m(E_POm, Ts, v_m, E_PCm_prev)

if (E_POm < 0 && v_m ~= 0)
    alpha_m = (-E_POm)/Ts*v_m^2;
else
    alpha_m = 0;
end

E_PCm = E_PCm_prev + (alpha_m*v_m^2)*Ts;

== matlab function PHRI_MODEL_PROJECT/MASTER SIDE1/Velocity Approx + LPF /Euler Approximation  ==
  data: beta input; Ts input; filtered output; pos input; posPrev input; filteredPrev input
function filtered = EulApprox(beta, Ts, pos, posPrev, filteredPrev)

eul= (pos - posPrev)/Ts;
filtered = beta*eul + (1-beta)*filteredPrev;

== matlab function PHRI_MODEL_PROJECT/POPC - Master Side1/PC - Master side/PASSIVE CONTROLLER PCm ==
  data: E_POm input; E_PCm output; dt input; v_m input; E_PCm_prev input; alpha_m output
function [E_PCm, alpha_m]= PC_m(E_POm, dt, v_m, E_PCm_prev)

if (E_POm < 0 && v_m ~= 0)
    alpha_m = (-E_POm)/dt*v_m^2;
else
    alpha_m = 0;
end

E_PCm = E_PCm_prev + (alpha_m*v_m^2)*dt;

== matlab function PHRI_MODEL_PROJECT/SLAVE_SIDE /Velocity Approx + LPF 1/Euler Approximation  ==
  data: beta input; Ts input; filtered output; pos input; posPrev input; filteredPrev input
function filtered = EulApprox(beta, Ts, pos, posPrev, filteredPrev)

eul= (pos - posPrev)/Ts;
filtered = beta*eul + (1-beta)*filteredPrev;

== matlab function PHRI_MODEL_PROJECT/POPC - Slave Side1/PC Slave/PASSIVE CONTROLLER PCs ==
  data: E_PCs_prev input; E_POs input; E_PCs output; Ts input; v_s input; alpha_s output
function [E_PCs, alpha_s]= PC_s(E_PCs_prev, E_POs, Ts, v_s)

if (E_POs < 0 && v_s ~= 0)
    alpha_s = (-E_POs)/Ts*v_s^2;
else
    alpha_s = 0;
end

E_PCs = E_PCs_prev + (alpha_s*v_s^2)*Ts;

== matlab function PHRI_MODEL_PROJECT/SLAVE_SIDE 1/Environment /Environment Behaviour ==
  data: x_s input; Fe output; dot_x_s input; qe input; Be input; Ke input
function Fe = Env(x_s, dot_x_s, qe, Be, Ke)
    
    if(x_s > qe)
        Fe = Ke*(x_s - qe) + Be*dot_x_s;
    else
        Fe = 0;
    end

== matlab function PHRI_MODEL_PROJECT/SLAVE_SIDE 1/Euler Approximation Vel MH1/Euler Approximation  ==
  data: beta input; Ts input; filtered output; pos input; posPrev input; filteredPrev input
function filtered = EulApprox(beta, Ts, pos, posPrev, filteredPrev)

eul= (pos - posPrev)/Ts;
filtered = beta*eul + (1-beta)*filteredPrev;

== matlab function PHRI_MODEL_PROJECT/SLAVE_SIDE 1/Velocity Approx + LPF /Euler Approximation  ==
  data: beta input; Ts input; filtered output; pos input; posPrev input; filteredPrev input
function filtered = EulApprox(beta, Ts, pos, posPrev, filteredPrev)

eul= (pos - posPrev)/Ts;
filtered = beta*eul + (1-beta)*filteredPrev;

== matlab function PHRI_MODEL_PROJECT/Euler Approximation Vel M2/Euler Approximation  ==
  data: beta input; Ts input; filtered output; pos input; posPrev input; filteredPrev input
function filtered = EulApprox(beta, Ts, pos, posPrev, filteredPrev)

eul= (pos - posPrev)/Ts;
filtered = beta*eul + (1-beta)*filteredPrev;

== matlab function PHRI_MODEL_PROJECT/MASTER SIDE2/Velocity Approx + LPF /Euler Approximation  ==
  data: beta input; Ts input; filtered output; pos input; posPrev input; filteredPrev input
function filtered = EulApprox(beta, Ts, pos, posPrev, filteredPrev)

eul= (pos - posPrev)/Ts;
filtered = beta*eul + (1-beta)*filteredPrev;

== matlab function PHRI_MODEL_PROJECT/MASTER SIDE2/Velocity Approx + LPF 1/Euler Approximation  ==
  data: beta input; Ts input; filtered output; pos input; posPrev input; filteredPrev input
function filtered = EulApprox(beta, Ts, pos, posPrev, filteredPrev)

eul= (pos - posPrev)/Ts;
filtered = beta*eul + (1-beta)*filteredPrev;

== matlab function PHRI_MODEL_PROJECT/SLAVE_SIDE /Environment /Environment Behaviour ==
  data: x_s input; Fe output; dot_x_s input; qe input; Be input; Ke input
function Fe = Env(x_s, dot_x_s, qe, Be, Ke)
    
    if(x_s > qe)
        Fe = Ke*(x_s - qe) + Be*dot_x_s;
    else
        Fe = 0;
    end

== matlab function PHRI_MODEL_PROJECT/MASTER SIDE2/Velocity Approx + LPF 2/Euler Approximation  ==
  data: beta input; Ts input; filtered output; pos input; posPrev input; filteredPrev input
function filtered = EulApprox(beta, Ts, pos, posPrev, filteredPrev)

eul= (pos - posPrev)/Ts;
filtered = beta*eul + (1-beta)*filteredPrev;

== matlab function PHRI_MODEL_PROJECT/MASTER SIDE2/Velocity Approx + LPF 3/Euler Approximation  ==
  data: beta input; Ts input; filtered output; pos input; posPrev input; filteredPrev input
function filtered = EulApprox(beta, Ts, pos, posPrev, filteredPrev)

eul= (pos - posPrev)/Ts;
filtered = beta*eul + (1-beta)*filteredPrev;

== matlab function PHRI_MODEL_PROJECT/Operator Stiffness2/Operator Stiffness  ==
  data: KhMax input; Kh input; Kh_func output; t input; stopTime input
function Kh_func = stiffness(KhMax, Kh, t, stopTime)
%Solving cubic polynomial function to model the operator stiffness
%(f'(begin) + f'(end) - 2*f(begin))(x/k)^3 + (3*f(end) - 2*f'(begin) - f'(end))(x/k)^2 + f'(begin)x/k + f(begin)

    begin = 0.5;

    endTime = stopTime-0.5;

    df_begin = 0;
    df_end = 0;
    f_end = KhMax - Kh;

    if t < begin
    Kh_func = Kh;
    else
    Kh_func = (df_begin + df_end - 2*f_end)*((t-begin)/endTime)^3 + (3*f_end - 2*df_begin - df_end)*((t-begin)/endTime)^2 + (df_begin)*((t-begin)/endTime) + Kh;
    end
end

== matlab function PHRI_MODEL_PROJECT/POPC - Master Side2/PC - Master side/PASSIVE CONTROLLER PCm ==
  data: E_POm input; E_PCm output; dt input; v_m input; E_PCm_prev input; alpha_m output
function [E_PCm, alpha_m]= PC_m(E_POm, dt, v_m, E_PCm_prev)

if (E_POm < 0 && v_m ~= 0)
    alpha_m = (-E_POm)/dt*v_m^2;
else
    alpha_m = 0;
end

E_PCm = E_PCm_prev + (alpha_m*v_m^2)*dt;

== matlab function PHRI_MODEL_PROJECT/POPC - Slave Side2/PC Slave/PASSIVE CONTROLLER PCs ==
  data: E_PCs_prev input; E_POs input; E_PCs output; Ts input; v_s input; alpha_s output
function [E_PCs, alpha_s]= PC_s(E_PCs_prev, E_POs, Ts, v_s)

if (E_POs < 0 && v_s ~= 0)
    alpha_s = (-E_POs)/Ts*v_s^2;
else
    alpha_s = 0;
end

E_PCs = E_PCs_prev + (alpha_s*v_s^2)*Ts;

== matlab function PHRI_MODEL_PROJECT/SLAVE_SIDE 2/Environment /Environment Behaviour ==
  data: x_s input; Fe output; dot_x_s input; qe input; Be input; Ke input
function Fe = Env(x_s, dot_x_s, qe, Be, Ke)
    
    if(x_s > qe)
        Fe = Ke*(x_s - qe) + Be*dot_x_s;
    else
        Fe = 0;
    end

== matlab function PHRI_MODEL_PROJECT/SLAVE_SIDE 2/Euler Approximation Vel MH1/Euler Approximation  ==
  data: beta input; Ts input; filtered output; pos input; posPrev input; filteredPrev input
function filtered = EulApprox(beta, Ts, pos, posPrev, filteredPrev)

eul= (pos - posPrev)/Ts;
filtered = beta*eul + (1-beta)*filteredPrev;

== matlab function PHRI_MODEL_PROJECT/SLAVE_SIDE 2/Velocity Approx + LPF /Euler Approximation  ==
  data: beta input; Ts input; filtered output; pos input; posPrev input; filteredPrev input
function filtered = EulApprox(beta, Ts, pos, posPrev, filteredPrev)

eul= (pos - posPrev)/Ts;
filtered = beta*eul + (1-beta)*filteredPrev;

== matlab function PHRI_MODEL_PROJECT/POPC - Slave Side/PC Slave/PASSIVE CONTROLLER PCs ==
  data: E_PCs_prev input; E_POs input; E_PCs output; Ts input; v_s input; alpha_s output
function [E_PCs, alpha_s]= PC_s(E_PCs_prev, E_POs, Ts, v_s)

if (E_POs < 0 && v_s ~= 0)
    alpha_s = (-E_POs)/Ts*v_s^2;
else
    alpha_s = 0;
end

E_PCs = E_PCs_prev + (alpha_s*v_s^2)*Ts;

== matlab function PHRI_MODEL_PROJECT/Operator Stiffness/Operator Stiffness  ==
  data: KhMax input; Kh input; Kh_func output; t input; stopTime input
function Kh_func = stiffness(KhMax, Kh, t, stopTime)
%Solving cubic polynomial function to model the operator stiffness
%(f'(begin) + f'(end) - 2*f(begin))(x/k)^3 + (3*f(end) - 2*f'(begin) - f'(end))(x/k)^2 + f'(begin)x/k + f(begin)

    begin = 0.5;

    endTime = stopTime-0.5;

    df_begin = 0;
    df_end = 0;
    f_end = KhMax - Kh;

    if t < begin
    Kh_func = Kh;
    else
    Kh_func = (df_begin + df_end - 2*f_end)*((t-begin)/endTime)^3 + (3*f_end - 2*df_begin - df_end)*((t-begin)/endTime)^2 + (df_begin)*((t-begin)/endTime) + Kh;
    end
end

== matlab function PHRI_MODEL_PROJECT/Operator Stiffness1/Operator Stiffness  ==
  data: KhMax input; Kh input; Kh_func output; t input; stopTime input
function Kh_func = stiffness(KhMax, Kh, t, stopTime)
%Solving cubic polynomial function to model the operator stiffness
%(f'(begin) + f'(end) - 2*f(begin))(x/k)^3 + (3*f(end) - 2*f'(begin) - f'(end))(x/k)^2 + f'(begin)x/k + f(begin)

    begin = 0.5;

    endTime = stopTime-0.5;

    df_begin = 0;
    df_end = 0;
    f_end = KhMax - Kh;

    if t < begin
    Kh_func = Kh;
    else
    Kh_func = (df_begin + df_end - 2*f_end)*((t-begin)/endTime)^3 + (3*f_end - 2*df_begin - df_end)*((t-begin)/endTime)^2 + (df_begin)*((t-begin)/endTime) + Kh;
    end
end
